simulink model "driver_interface"  (R2022b)
settings: Solver=FixedStepAuto  StartTime=0.0  StopTime=10.0  RelTol=1e-3
libraries: driver_interface_lib x8
settings Model: Creator=dr_pa  LastModifiedBy=dr_pa
settings OptimizationCC: DefaultParameterBehavior=Inlined  EnhancedBackFolding=on  PassReuseOutputArgsAs=Individual arguments  ZeroExternalMemoryAtStartup=off  ZeroInternalMemoryAtStartup=off  OptimizeBlockOrder=speed  DifferentSizesBufferReuse=on  OptimizationCustomize=off  EfficientTunableParamExpr=on
settings DebuggingCC: ParameterTunabilityLossMsg=error
settings SFSimCC: MATLABDynamicMemAlloc=off
settings RTWCC: Description=Embedded Coder  SystemTargetFile=ert.tlc  GenCodeOnly=on  TemplateMakefile=ert_default_tmf
settings CodeAppCC: ForceParamTrailComments=on  IgnoreCustomStorageClasses=off  OperatorAnnotations=on  SimulinkDataObjDesc=on  SFDataObjDesc=on  InsertBlockDesc=on
settings ERTTargetCC: TargetLangStandard=C99 (ISO)  GenerateSampleERTMain=on  InlinedParameterPlacement=NonHierarchical  ERTCustomFileTemplate=example_file_process.tlc

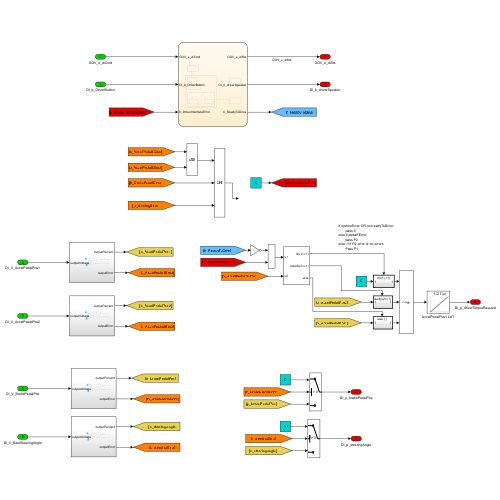
[thumbnail: Simulink's stored preview of the top-level diagram]
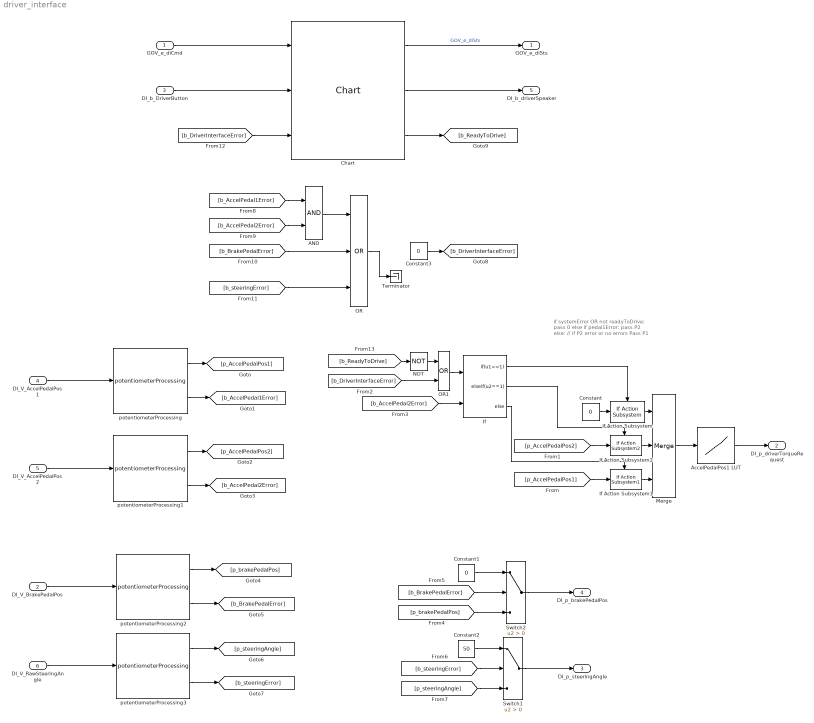
== system driver_interface ==
  note: if systemError OR not readyToDrive:
      | 	pass 0
      | else if pedal1Error:
      | 	pass P2
      | else: // if P2 error or no errors
      | 	Pass P1
  GOV_e_diCmd : Inport
  DI_V_BrakePedalPos : Inport  Port=2
  DI_b_DriverButton : Inport  Port=3
  DI_V_AccelPedalPos1 : Inport  Port=4
  DI_V_AccelPedalPos2 : Inport  Port=5
  Dl_V_RawSteeringAngle : Inport  Port=6
  AND : Logic  AllPortsSameDT=off  OutDataTypeStr=boolean
  AccelPedalPos1 LUT : Lookup_n-D  NumberOfTableDimensions=1  BreakpointsForDimension1=[0 5 10 15 20 25 30 35 40 45 50 55 60 65 70 75 80 85 90 95 100]  Table=[0 5 10 15 20 25 30 35 40 45 50 55 60 65 70 75 80 85 90 95 100]  InternalRulePriority=Speed  RndMeth=Simplest
  Chart : driver_interface_lib/driver_interface/Chart  SystemSampleTime=-1  VariantActivationTime=update diagram  Latency=0  AutoFrameSizeCalculation=off
  Constant : Constant  Value=0  OutDataTypeStr=single
  Constant1 : Constant  Value=0  OutDataTypeStr=single
  Constant2 : Constant  Value=50  OutDataTypeStr=single
  Constant3 : Constant  Value=0  OutDataTypeStr=boolean
  If : If  NumInputs=2  IfExpression=u1==1  ElseIfExpressions=u2==1
  If Action Subsystem : driver_interface_lib/driver_interface/If Action Subsystem  SystemSampleTime=-1  VariantActivationTime=update diagram  Latency=0  AutoFrameSizeCalculation=off
  If Action Subsystem1 : driver_interface_lib/driver_interface/If Action Subsystem1  SystemSampleTime=-1  VariantActivationTime=update diagram  Latency=0  AutoFrameSizeCalculation=off
  If Action Subsystem2 : driver_interface_lib/driver_interface/If Action Subsystem2  SystemSampleTime=-1  VariantActivationTime=update diagram  Latency=0  AutoFrameSizeCalculation=off
  Merge : Merge  Inputs=3
  NOT : Logic  Operator=NOT  IconShape=distinctive  AllPortsSameDT=off  OutDataTypeStr=boolean
  OR : Logic  Operator=OR  Inputs=3  AllPortsSameDT=off  OutDataTypeStr=boolean
  OR1 : Logic  Operator=OR  AllPortsSameDT=off  OutDataTypeStr=boolean
  Switch1 : Switch  Criteria=u2 > Threshold  SaturateOnIntegerOverflow=off  InputSameDT=off
  Switch2 : Switch  Criteria=u2 > Threshold  SaturateOnIntegerOverflow=off  InputSameDT=off
  Terminator : Terminator
  potentiometerProcessing{,1..3} (4 alike) : driver_interface_lib/driver_interface/potentiometerProcessing  SystemSampleTime=-1  VariantActivationTime=update diagram  Latency=0  AutoFrameSizeCalculation=off
  GOV_e_diSts : Outport
  DI_p_driverTorqueRequest : Outport  Port=2
  DI_p_steeringAngle : Outport  Port=3
  DI_p_brakePedalPos : Outport  Port=4
  DI_b_driverSpeaker : Outport  Port=5
  wires:
  potentiometerProcessing/2 -> [b_AccelPedal1Error]
  Merge/1 -> AccelPedalPos1 LUT/1
  AccelPedalPos1 LUT/1 -> DI_p_driverTorqueRequest/1
  DI_V_AccelPedalPos1/1 -> potentiometerProcessing/1
  potentiometerProcessing2/1 -> [p_brakePedalPos]
  If Action Subsystem1/1 -> Merge/3
  potentiometerProcessing1/1 -> [p_AccelPedalPos2]
  potentiometerProcessing1/2 -> [b_AccelPedal2Error]
  If Action Subsystem2/1 -> Merge/2
  [b_steeringError] -> OR/3
  GOV_e_diCmd/1 -> Chart/1
  Dl_V_RawSteeringAngle/1 -> potentiometerProcessing3/1
  potentiometerProcessing3/1 -> [p_steeringAngle]
  [p_steeringAngle] -> Switch1/3
  [b_steeringError] -> Switch1/2
  [p_AccelPedalPos1] -> If Action Subsystem1/1
  DI_V_BrakePedalPos/1 -> potentiometerProcessing2/1
  [b_AccelPedal2Error] -> AND/2
  If/3 -> If Action Subsystem1/Action
  OR1/1 -> If/1
  Constant/1 -> If Action Subsystem/1
  DI_b_DriverButton/1 -> Chart/2
  Chart/3 -> [b_ReadyToDrive]
  Chart/1 -> GOV_e_diSts/1  "GOV_e_diSts"
  [b_DriverInterfaceError] -> Chart/3
  potentiometerProcessing3/2 -> [b_steeringError]
  Chart/2 -> DI_b_driverSpeaker/1
  AND/1 -> OR/1
  [p_AccelPedalPos2] -> If Action Subsystem2/1
  potentiometerProcessing/1 -> [p_AccelPedalPos1]
  [b_BrakePedalError] -> Switch2/2
  If/1 -> If Action Subsystem/Action
  Switch2/1 -> DI_p_brakePedalPos/1
  [b_AccelPedal1Error] -> AND/1
  If Action Subsystem/1 -> Merge/1
  potentiometerProcessing2/2 -> [b_BrakePedalError]
  Constant3/1 -> [b_DriverInterfaceError]
  DI_V_AccelPedalPos2/1 -> potentiometerProcessing1/1
  [p_brakePedalPos] -> Switch2/3
  [b_DriverInterfaceError] -> OR1/2
  OR/1 -> Terminator/1
  Constant1/1 -> Switch2/1
  NOT/1 -> OR1/1
  Constant2/1 -> Switch1/1
  [b_BrakePedalError] -> OR/2
  If/2 -> If Action Subsystem2/Action
  [b_AccelPedal2Error] -> If/2
  Switch1/1 -> DI_p_steeringAngle/1
  [b_ReadyToDrive] -> NOT/1
